simulink model "DataAcquire"  (R2017a)
settings: Solver=FixedStepDiscrete  StartTime=0.0  StopTime=inf  RelTol=1e-3  EnableMultiTasking=on
libraries: simulink x54, stmmbedlib x40
settings Model: SimulationMode=external  ExtModeArchiveFileName=LOGGING  ExtModeArchiveDirName=C:\Users\Salokin\Dropbox\StudiumJobs\Fahrrad Hiwi\STMDISCO  ExtModeAutoIncOneShot=on  Creator=The MathWorks, Inc.  LastModifiedBy=Salokin
settings DataIOCC: LimitDataPoints=on  SaveFormat=Array
settings OptimizationCC: LifeSpan=Inf  MaxStackSize=64
settings DebuggingCC: UnderspecifiedInitializationDetection=Classic  MergeDetectMultiDrivingBlocksExec=none  SolverPrmCheckMsg=warning  AllowSymbolicDim=off  SFUnexpectedBacktrackingDiag=warning  SFNoUnconditionalDefaultTransitionDiag=warning  SFExecutionAtInitializationDiag=none
settings HardwareCC: ProdBitPerPointer=32  ProdBitPerSizeT=32  ProdBitPerPtrDiffT=32  ProdLargestAtomicInteger=Long  ProdLargestAtomicFloat=Double  ProdWordSize=32  ProdHWDeviceType=ARM Compatible->ARM Cortex
settings ModelReferenceCC: PropagateSignalLabelsOutOfModel=off
settings SFSimCC: MATLABDynamicMemAlloc=off
settings RTWCC: SystemTargetFile=ert.tlc  HardwareBoard=STM32F746G-Discovery  TemplateMakefile=ert_default_tmf  Description=Embedded Coder  Toolchain=GNU Tools for ARM Embedded Processors
settings CodeAppCC: IgnoreCustomStorageClasses=off  CustomSymbolStrModelFcn=$N
settings ERTTargetCC: MultiwordLength=2048  ExtMode=on  ExtModeTransport=1  ExtModeMexFile=ext_serial_win32_comm  ExtModeMexArgs=0 28 460800  ConvertIfToSwitch=off  SuppressUnreachableDefaultCases=off
settings ConfigComp: CovMetricSettings=dw  CovHtmlReporting=on  CovSaveCumulativeToWorkspaceVar=on  CovSaveSingleToWorkspaceVar=on  CovExternalEMLEnable=off  CovSFcnEnable=off

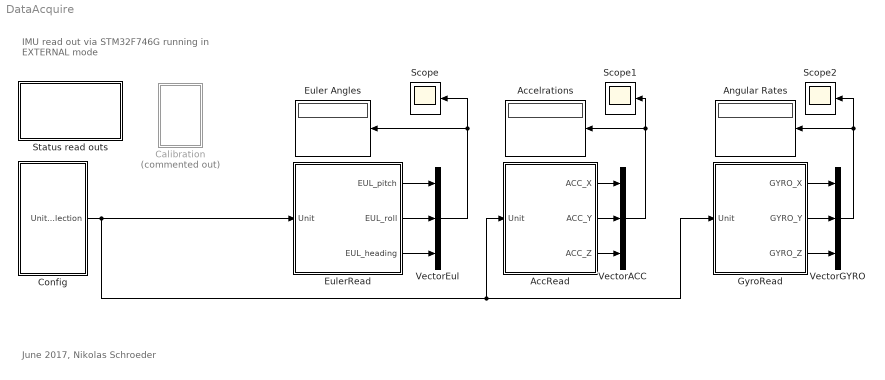
== system DataAcquire ==
  note: June 2017, Nikolas Schroeder
  note: IMU read out via STM32F746G
      | running in EXTERNAL mode
  AccRead : Subsystem
  Accelrations : Display
  Angular Rates : Display
  Calibration : Subsystem  Commented=on
  Config : Subsystem
  Euler Angles : Display
  EulerRead : Subsystem
  GyroRead : Subsystem
  Scope : Scope
  Scope1 : Scope
  Scope2 : Scope
  Status read outs : Subsystem
  VectorACC : Concatenate  NumInputs=3
  VectorEul : Concatenate  NumInputs=3
  VectorGYRO : Concatenate  NumInputs=3
  wires:
  AccRead/1(ACC_X) -> VectorACC/1
  AccRead/2(ACC_Y) -> VectorACC/2
  AccRead/3(ACC_Z) -> VectorACC/3
  GyroRead/1(GYRO_X) -> VectorGYRO/1
  GyroRead/2(GYRO_Y) -> VectorGYRO/2
  GyroRead/3(GYRO_Z) -> VectorGYRO/3
  VectorACC/1 -> Accelrations/1, Scope1/1
  VectorGYRO/1 -> Scope2/1, Angular Rates/1
  EulerRead/1(EUL_pitch) -> VectorEul/1
  EulerRead/2(EUL_roll) -> VectorEul/2
  EulerRead/3(EUL_heading) -> VectorEul/3
  VectorEul/1 -> Scope/1, Euler Angles/1
  Config/1(UnitSelection) -> GyroRead/1(Unit), AccRead/1(Unit), EulerRead/1(Unit)

== system DataAcquire/AccRead ==
  Unit : Inport
  ACCEL_Data_X1_MSB : stmmbedlib/I2C Master Read  I2CModule=0  Mode=Master  SlaveAddress=hex2dec('28')  SlaveByteOrder=BigEndian  Direction=Receiver  RegisterAddressMode=on  RegisterAddress=hex2dec('09')  SlaveDataType=uint8  DataLength=1  NoAck=off  RepeatedStart=off  OutputStatus=on  SampleTime=0.1
  ACCEL_Data_X_LSB : stmmbedlib/I2C Master Read  I2CModule=0  Mode=Master  SlaveAddress=hex2dec('28')  SlaveByteOrder=BigEndian  Direction=Receiver  RegisterAddressMode=on  RegisterAddress=hex2dec('08')  SlaveDataType=uint8  DataLength=1  NoAck=off  RepeatedStart=off  OutputStatus=on  SampleTime=0.1
  ACCEL_Data_Y1_MSB : stmmbedlib/I2C Master Read  I2CModule=0  Mode=Master  SlaveAddress=hex2dec('28')  SlaveByteOrder=BigEndian  Direction=Receiver  RegisterAddressMode=on  RegisterAddress=hex2dec('0B')  SlaveDataType=uint8  DataLength=1  NoAck=off  RepeatedStart=off  OutputStatus=on  SampleTime=0.1
  "ACCEL_Data_Y_LSB " : stmmbedlib/I2C Master Read  I2CModule=0  Mode=Master  SlaveAddress=hex2dec('28')  SlaveByteOrder=BigEndian  Direction=Receiver  RegisterAddressMode=on  RegisterAddress=hex2dec('0A')  SlaveDataType=uint8  DataLength=1  NoAck=off  RepeatedStart=off  OutputStatus=on  SampleTime=0.1
  ACCEL_Data_Z1_MSB : stmmbedlib/I2C Master Read  I2CModule=0  Mode=Master  SlaveAddress=hex2dec('28')  SlaveByteOrder=BigEndian  Direction=Receiver  RegisterAddressMode=on  RegisterAddress=hex2dec('0D')  SlaveDataType=uint8  DataLength=1  NoAck=off  RepeatedStart=off  OutputStatus=on  SampleTime=0.1
  ACCEL_Data_Z_LSB : stmmbedlib/I2C Master Read  I2CModule=0  Mode=Master  SlaveAddress=hex2dec('28')  SlaveByteOrder=BigEndian  Direction=Receiver  RegisterAddressMode=on  RegisterAddress=hex2dec('0C')  SlaveDataType=uint8  DataLength=1  NoAck=off  RepeatedStart=off  OutputStatus=on  SampleTime=0.1
  ACCparserX : Subsystem
  ACCparserY : Subsystem
  ACCparserZ : Subsystem
  Error Status{,1..5} (6 alike) : Display
  ACC_X : Outport
  ACC_Y : Outport  Port=2
  ACC_Z : Outport  Port=3
  wires:
  "ACCEL_Data_Y_LSB "/2 -> Error Status3/1
  ACCEL_Data_Y1_MSB/2 -> Error Status2/1
  ACCEL_Data_Z1_MSB/1 -> ACCparserZ/2(MSB)
  ACCEL_Data_X_LSB/2 -> Error Status/1
  "ACCEL_Data_Y_LSB "/1 -> ACCparserY/1(LSB)
  ACCEL_Data_X1_MSB/2 -> Error Status1/1
  ACCEL_Data_Z_LSB/2 -> Error Status4/1
  ACCEL_Data_Y1_MSB/1 -> ACCparserY/2(MSB)
  ACCEL_Data_Z1_MSB/2 -> Error Status5/1
  ACCEL_Data_Z_LSB/1 -> ACCparserZ/1(LSB)
  Unit/1 -> ACCparserX/3(Unit), ACCparserZ/3(Unit), ACCparserY/3(Unit)
  ACCparserX/1(Out1) -> ACC_X/1
  ACCparserY/1(Out1) -> ACC_Y/1
  ACCEL_Data_X1_MSB/1 -> ACCparserX/2(MSB)
  ACCEL_Data_X_LSB/1 -> ACCparserX/1(LSB)
  ACCparserZ/1(Out1) -> ACC_Z/1

== system DataAcquire/Calibration ==
  Constant{,1..3} (4 alike) : Constant
  I2C Master Write{,1..3} (4 alike) : stmmbedlib/I2C Master Write  I2CModule=0  Mode=Master  SlaveAddress=hex2dec('48')  SlaveByteOrder=BigEndian  Direction=Transmitter  RegisterAddressMode=on  RegisterAddress=uint8(1)  SlaveDataType=uint8  DataLength=2  NoAck=off  RepeatedStart=off  OutputStatus=off
  wires:
  Constant/1 -> I2C Master Write3/1
  Constant2/1 -> I2C Master Write1/1
  Constant3/1 -> I2C Master Write/1
  Constant1/1 -> I2C Master Write2/1

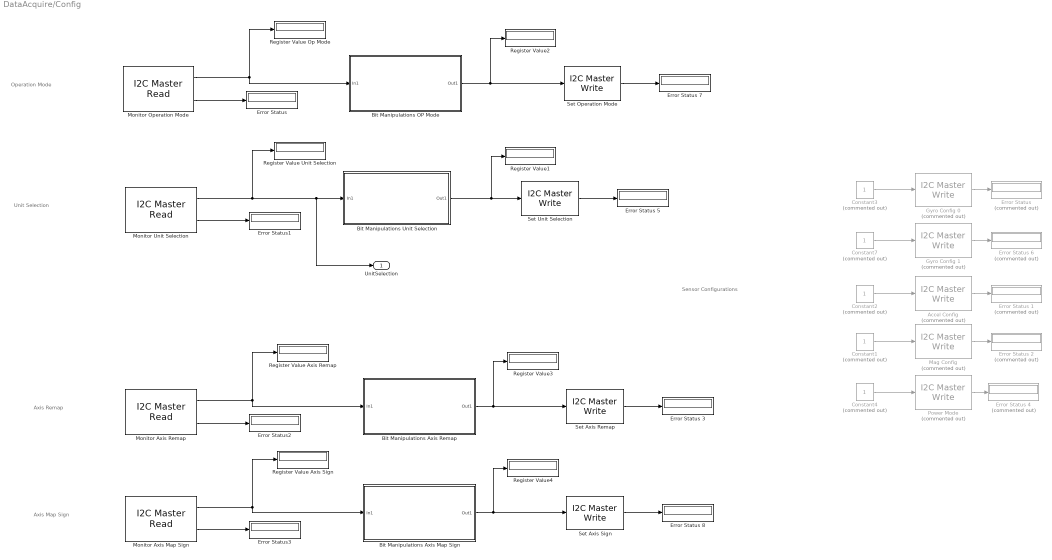
== system DataAcquire/Config ==
  note: Unit Selection
  note: Operation Mode
  note: Sensor Configurations
  note: Axis Remap
  note: Axis Map Sign
  Accel Config : stmmbedlib/I2C Master Write  Commented=on  I2CModule=0  Mode=Master  SlaveAddress=hex2dec('28')  SlaveByteOrder=BigEndian  Direction=Transmitter  RegisterAddressMode=on  RegisterAddress=hex2dec('8')  SlaveDataType=uint8  DataLength=2  NoAck=off  RepeatedStart=off  OutputStatus=on
  Bit Manipulations Axis Map Sign : Subsystem
  Bit Manipulations Axis Remap : Subsystem
  Bit Manipulations OP Mode : Subsystem
  Bit Manipulations Unit Selection : Subsystem
  Constant{1..4,7} (5 alike) : Constant  Commented=on
  Error Status{,1..3} (4 alike) : Display
  Error Status {,1..2,4,6} (5 alike) : Display  Commented=on
  Error Status {3,5,7..8} (4 alike) : Display
  Gyro Config 0 : stmmbedlib/I2C Master Write  Commented=on  I2CModule=0  Mode=Master  SlaveAddress=hex2dec('28')  SlaveByteOrder=BigEndian  Direction=Transmitter  RegisterAddressMode=on  RegisterAddress=hex2dec('A')  SlaveDataType=uint8  DataLength=2  NoAck=off  RepeatedStart=off  OutputStatus=on
  Gyro Config 1 : stmmbedlib/I2C Master Write  Commented=on  I2CModule=0  Mode=Master  SlaveAddress=hex2dec('28')  SlaveByteOrder=BigEndian  Direction=Transmitter  RegisterAddressMode=on  RegisterAddress=hex2dec('B')  SlaveDataType=uint8  DataLength=2  NoAck=off  RepeatedStart=off  OutputStatus=on
  Mag Config : stmmbedlib/I2C Master Write  Commented=on  I2CModule=0  Mode=Master  SlaveAddress=hex2dec('28')  SlaveByteOrder=BigEndian  Direction=Transmitter  RegisterAddressMode=on  RegisterAddress=hex2dec('9')  SlaveDataType=uint8  DataLength=2  NoAck=off  RepeatedStart=off  OutputStatus=on
  Monitor Axis Map Sign : stmmbedlib/I2C Master Read  I2CModule=0  Mode=Master  SlaveAddress=hex2dec('28')  SlaveByteOrder=BigEndian  Direction=Receiver  RegisterAddressMode=on  RegisterAddress=hex2dec('42')  SlaveDataType=uint8  DataLength=1  NoAck=off  RepeatedStart=off  OutputStatus=on  SampleTime=0.1
  Monitor Axis Remap : stmmbedlib/I2C Master Read  I2CModule=0  Mode=Master  SlaveAddress=hex2dec('28')  SlaveByteOrder=BigEndian  Direction=Receiver  RegisterAddressMode=on  RegisterAddress=hex2dec('41')  SlaveDataType=uint8  DataLength=1  NoAck=off  RepeatedStart=off  OutputStatus=on  SampleTime=0.1
  Monitor Operation Mode : stmmbedlib/I2C Master Read  I2CModule=0  Mode=Master  SlaveAddress=hex2dec('28')  SlaveByteOrder=BigEndian  Direction=Receiver  RegisterAddressMode=on  RegisterAddress=hex2dec('3d')  SlaveDataType=uint8  DataLength=1  NoAck=off  RepeatedStart=off  OutputStatus=on  SampleTime=0.01
  Monitor Unit Selection : stmmbedlib/I2C Master Read  I2CModule=0  Mode=Master  SlaveAddress=hex2dec('28')  SlaveByteOrder=BigEndian  Direction=Receiver  RegisterAddressMode=on  RegisterAddress=hex2dec('3b')  SlaveDataType=uint8  DataLength=1  NoAck=off  RepeatedStart=off  OutputStatus=on  SampleTime=0.1
  Power Mode : stmmbedlib/I2C Master Write  Commented=on  I2CModule=0  Mode=Master  SlaveAddress=hex2dec('28')  SlaveByteOrder=BigEndian  Direction=Transmitter  RegisterAddressMode=on  RegisterAddress=hex2dec('3E')  SlaveDataType=uint8  DataLength=2  NoAck=off  RepeatedStart=off  OutputStatus=on
  Register Value Axis Remap : Display
      settings: Format=binary (Stored Integer)
  Register Value Axis Sign : Display
      settings: Format=binary (Stored Integer)
  "Register Value Op Mode " : Display
      settings: Format=binary (Stored Integer)
  Register Value Unit Selection : Display
      settings: Format=binary (Stored Integer)
  Register Value{1..4} (4 alike) : Display
      settings: Format=binary (Stored Integer)
  Set Axis Remap : stmmbedlib/I2C Master Write  I2CModule=0  Mode=Master  SlaveAddress=hex2dec('28')  SlaveByteOrder=BigEndian  Direction=Transmitter  RegisterAddressMode=on  RegisterAddress=hex2dec('41')  SlaveDataType=uint8  DataLength=2  NoAck=off  RepeatedStart=off  OutputStatus=on
  Set Axis Sign : stmmbedlib/I2C Master Write  I2CModule=0  Mode=Master  SlaveAddress=hex2dec('28')  SlaveByteOrder=BigEndian  Direction=Transmitter  RegisterAddressMode=on  RegisterAddress=hex2dec('42')  SlaveDataType=uint8  DataLength=2  NoAck=off  RepeatedStart=off  OutputStatus=on
  Set Operation Mode : stmmbedlib/I2C Master Write  I2CModule=0  Mode=Master  SlaveAddress=hex2dec('28')  SlaveByteOrder=BigEndian  Direction=Transmitter  RegisterAddressMode=on  RegisterAddress=hex2dec('3D')  SlaveDataType=uint8  DataLength=2  NoAck=off  RepeatedStart=off  OutputStatus=on
  Set Unit Selection : stmmbedlib/I2C Master Write  I2CModule=0  Mode=Master  SlaveAddress=hex2dec('28')  SlaveByteOrder=BigEndian  Direction=Transmitter  RegisterAddressMode=on  RegisterAddress=hex2dec('3b')  SlaveDataType=uint8  DataLength=2  NoAck=off  RepeatedStart=off  OutputStatus=on
  UnitSelection : Outport
  wires:
  Constant2/1 -> Accel Config/1
  Constant3/1 -> Gyro Config 0/1
  Constant1/1 -> Mag Config/1
  Constant4/1 -> Power Mode/1
  Gyro Config 0/1 -> "Error Status "/1
  Accel Config/1 -> Error Status 1/1
  Mag Config/1 -> Error Status 2/1
  Power Mode/1 -> Error Status 4/1
  Constant7/1 -> Gyro Config 1/1
  Gyro Config 1/1 -> Error Status 6/1
  Monitor Operation Mode/2 -> Error Status/1
  Monitor Operation Mode/1 -> "Register Value Op Mode "/1, Bit Manipulations OP Mode/1(In1)
  Set Operation Mode/1 -> Error Status 7/1
  Set Unit Selection/1 -> Error Status 5/1
  Monitor Unit Selection/1 -> UnitSelection/1, Bit Manipulations Unit Selection/1(In1), Register Value Unit Selection/1
  Monitor Unit Selection/2 -> Error Status1/1
  Bit Manipulations Unit Selection/1(Out1) -> Register Value1/1, Set Unit Selection/1
  Bit Manipulations OP Mode/1(Out1) -> Register Value2/1, Set Operation Mode/1
  Set Axis Sign/1 -> Error Status 8/1
  Bit Manipulations Axis Remap/1(Out1) -> Register Value3/1, Set Axis Remap/1
  Monitor Axis Remap/1 -> Register Value Axis Remap/1, Bit Manipulations Axis Remap/1(In1)
  Set Axis Remap/1 -> Error Status 3/1
  Monitor Axis Remap/2 -> Error Status2/1
  Monitor Axis Map Sign/1 -> Register Value Axis Sign/1, Bit Manipulations Axis Map Sign/1(In1)
  Monitor Axis Map Sign/2 -> Error Status3/1
  Bit Manipulations Axis Map Sign/1(Out1) -> Register Value4/1, Set Axis Sign/1

== system DataAcquire/EulerRead ==
  Unit : Inport
  EUL_Heading_LSB : stmmbedlib/I2C Master Read  I2CModule=0  Mode=Master  SlaveAddress=hex2dec('28')  SlaveByteOrder=BigEndian  Direction=Receiver  RegisterAddressMode=on  RegisterAddress=hex2dec('1A')  SlaveDataType=uint8  DataLength=1  NoAck=off  RepeatedStart=off  OutputStatus=on  SampleTime=0.1
  EUL_Heading_MSB : stmmbedlib/I2C Master Read  I2CModule=0  Mode=Master  SlaveAddress=hex2dec('28')  SlaveByteOrder=BigEndian  Direction=Receiver  RegisterAddressMode=on  RegisterAddress=hex2dec('1B')  SlaveDataType=uint8  DataLength=1  NoAck=off  RepeatedStart=off  OutputStatus=on  SampleTime=0.1
  "EUL_Pitch_LSB " : stmmbedlib/I2C Master Read  I2CModule=0  Mode=Master  SlaveAddress=hex2dec('28')  SlaveByteOrder=BigEndian  Direction=Receiver  RegisterAddressMode=on  RegisterAddress=hex2dec('1E')  SlaveDataType=uint8  DataLength=1  NoAck=off  RepeatedStart=off  OutputStatus=on  SampleTime=0.1
  "EUL_Pitch_MSB " : stmmbedlib/I2C Master Read  I2CModule=0  Mode=Master  SlaveAddress=hex2dec('28')  SlaveByteOrder=BigEndian  Direction=Receiver  RegisterAddressMode=on  RegisterAddress=hex2dec('1F')  SlaveDataType=uint8  DataLength=1  NoAck=off  RepeatedStart=off  OutputStatus=on  SampleTime=0.1
  "EUL_Roll_LSB " : stmmbedlib/I2C Master Read  I2CModule=0  Mode=Master  SlaveAddress=hex2dec('28')  SlaveByteOrder=BigEndian  Direction=Receiver  RegisterAddressMode=on  RegisterAddress=hex2dec('1C')  SlaveDataType=uint8  DataLength=1  NoAck=off  RepeatedStart=off  OutputStatus=on  SampleTime=0.1
  EUL_Roll_MSB : stmmbedlib/I2C Master Read  I2CModule=0  Mode=Master  SlaveAddress=hex2dec('28')  SlaveByteOrder=BigEndian  Direction=Receiver  RegisterAddressMode=on  RegisterAddress=hex2dec('1D')  SlaveDataType=uint8  DataLength=1  NoAck=off  RepeatedStart=off  OutputStatus=on  SampleTime=0.1
  EULparserHeading : Subsystem
  EULparserPitch : Subsystem
  EULparserRoll : Subsystem
  Error Status{,1..5} (6 alike) : Display
  EUL_pitch : Outport
  EUL_roll : Outport  Port=2
  EUL_heading : Outport  Port=3
  wires:
  EUL_Roll_MSB/2 -> Error Status2/1
  "EUL_Roll_LSB "/2 -> Error Status3/1
  "EUL_Roll_LSB "/1 -> EULparserRoll/1(LSB)
  EUL_Roll_MSB/1 -> EULparserRoll/2(MSB)
  EUL_Heading_MSB/2 -> Error Status5/1
  EUL_Heading_LSB/2 -> Error Status4/1
  EUL_Heading_LSB/1 -> EULparserHeading/1(LSB)
  EUL_Heading_MSB/1 -> EULparserHeading/2(MSB)
  "EUL_Pitch_MSB "/2 -> Error Status1/1
  "EUL_Pitch_MSB "/1 -> EULparserPitch/2(MSB)
  "EUL_Pitch_LSB "/2 -> Error Status/1
  "EUL_Pitch_LSB "/1 -> EULparserPitch/1(LSB)
  Unit/1 -> EULparserPitch/3(Unit), EULparserHeading/3(Unit), EULparserRoll/3(Unit)
  EULparserPitch/1(Out1) -> EUL_pitch/1
  EULparserRoll/1(Out1) -> EUL_roll/1
  EULparserHeading/1(Out1) -> EUL_heading/1

== system DataAcquire/GyroRead ==
  Unit : Inport
  Error Status{,1..5} (6 alike) : Display
  GYROparserX : Subsystem
  GYROparserY : Subsystem
  GYROparserZ : Subsystem
  Gyro_Data_X_LSB : stmmbedlib/I2C Master Read  I2CModule=0  Mode=Master  SlaveAddress=hex2dec('28')  SlaveByteOrder=BigEndian  Direction=Receiver  RegisterAddressMode=on  RegisterAddress=hex2dec('14')  SlaveDataType=uint8  DataLength=1  NoAck=off  RepeatedStart=off  OutputStatus=on  SampleTime=0.1
  Gyro_Data_X_MSB : stmmbedlib/I2C Master Read  I2CModule=0  Mode=Master  SlaveAddress=hex2dec('28')  SlaveByteOrder=BigEndian  Direction=Receiver  RegisterAddressMode=on  RegisterAddress=hex2dec('15')  SlaveDataType=uint8  DataLength=1  NoAck=off  RepeatedStart=off  OutputStatus=on  SampleTime=0.1
  Gyro_Data_Y_LSB : stmmbedlib/I2C Master Read  I2CModule=0  Mode=Master  SlaveAddress=hex2dec('28')  SlaveByteOrder=BigEndian  Direction=Receiver  RegisterAddressMode=on  RegisterAddress=hex2dec('16')  SlaveDataType=uint8  DataLength=1  NoAck=off  RepeatedStart=off  OutputStatus=on  SampleTime=0.1
  Gyro_Data_Y_MSB : stmmbedlib/I2C Master Read  I2CModule=0  Mode=Master  SlaveAddress=hex2dec('28')  SlaveByteOrder=BigEndian  Direction=Receiver  RegisterAddressMode=on  RegisterAddress=hex2dec('17')  SlaveDataType=uint8  DataLength=1  NoAck=off  RepeatedStart=off  OutputStatus=on  SampleTime=0.1
  Gyro_Data_Z_LSB : stmmbedlib/I2C Master Read  I2CModule=0  Mode=Master  SlaveAddress=hex2dec('28')  SlaveByteOrder=BigEndian  Direction=Receiver  RegisterAddressMode=on  RegisterAddress=hex2dec('18')  SlaveDataType=uint8  DataLength=1  NoAck=off  RepeatedStart=off  OutputStatus=on  SampleTime=0.1
  Gyro_Data_Z_MSB : stmmbedlib/I2C Master Read  I2CModule=0  Mode=Master  SlaveAddress=hex2dec('28')  SlaveByteOrder=BigEndian  Direction=Receiver  RegisterAddressMode=on  RegisterAddress=hex2dec('19')  SlaveDataType=uint8  DataLength=1  NoAck=off  RepeatedStart=off  OutputStatus=on  SampleTime=0.1
  GYRO_X : Outport
  GYRO_Y : Outport  Port=2
  GYRO_Z : Outport  Port=3
  wires:
  Gyro_Data_Z_MSB/1 -> GYROparserZ/2(MSB)
  Gyro_Data_X_LSB/2 -> Error Status/1
  Gyro_Data_X_MSB/2 -> Error Status1/1
  Gyro_Data_Z_LSB/2 -> Error Status4/1
  Gyro_Data_Y_LSB/2 -> Error Status3/1
  Gyro_Data_Z_LSB/1 -> GYROparserZ/1(LSB)
  Gyro_Data_Y_MSB/1 -> GYROparserY/2(MSB)
  Gyro_Data_Z_MSB/2 -> Error Status5/1
  Gyro_Data_Y_LSB/1 -> GYROparserY/1(LSB)
  GYROparserY/1(Out1) -> GYRO_Y/1
  Gyro_Data_Y_MSB/2 -> Error Status2/1
  Unit/1 -> GYROparserX/3(Unit), GYROparserZ/3(Unit), GYROparserY/3(Unit)
  GYROparserX/1(Out1) -> GYRO_X/1
  Gyro_Data_X_MSB/1 -> GYROparserX/2(MSB)
  Gyro_Data_X_LSB/1 -> GYROparserX/1(LSB)
  GYROparserZ/1(Out1) -> GYRO_Z/1

== system DataAcquire/Status read outs ==
  note: SYS_STATUS 0x39
      |
      | code (decimal)
      | content
      |
      | 0
      | System idle
      |
      | 1
      | System error
      |
      | 2
      | Initializing perpherals
      |
      | 3
      | System Initialization
      |
      | 4
      | Executing Self Test
      |
      | 5
      | Sensor Fusion Algorithm Running
      |
      | 6
      | System Running without fusion algorithm
  note: CALIB_STAT 0x35: 00 -> not calibrated, 11 -> calibrated
      |
      | bit
      | 7
      | 6
      | 5
      | 4
      | 3
      | 2
      | 1
      | 0
      |
      | content
      | SYS
      | GYRO
      | ACC
      | MAG
  note: ST_Result 0x36: 0 indicates failed Self Test, 1 indicates passed Self Test
      |
      | bit
      | 7 to 4
      | 3
      | 2
      | 1
      | 0
      |
      | content
      | reserved
      | Self Test result MCU
      | Self Test Result GYRO
      | Self Test result MAG
      | Self Test result ACC
  note: SYS_ERROR 0x3A
      |
      | error code (decimal)
      | content
      |
      | 0
      | No error
      |
      | 1
      | Peripheral initialization error
      |
      | 2
      | System initialization error
      |
      | 3
      | Self test result error
      |
      | 4
      | Register Map value out of range
      |
      | 5
      | Register Map address out of range
      |
      | 6
      | Register Map write error
      |
      | 7
      | BNO low power mode not available for selected operation mode
      |
      | 8
      | ACC power mode not available
      |
      | 9
      | Fusion mode configuration error
      |
      | 10
      | Sensor configuration error
  Calibration Status : stmmbedlib/I2C Master Read  Priority=2  I2CModule=0  Mode=Master  SlaveAddress=hex2dec('28')  SlaveByteOrder=BigEndian  Direction=Receiver  RegisterAddressMode=on  RegisterAddress=hex2dec('35')  SlaveDataType=uint8  DataLength=1  NoAck=off  RepeatedStart=off  OutputStatus=on  SampleTime=0.1
  Error Status{,1..4} (5 alike) : Display
  "Read out BNO055 Chip ID " : stmmbedlib/I2C Master Read  Priority=1  I2CModule=0  Mode=Master  SlaveAddress=hex2dec('28')  SlaveByteOrder=BigEndian  Direction=Receiver  RegisterAddressMode=on  RegisterAddress=hex2dec('00')  SlaveDataType=uint8  DataLength=1  NoAck=off  RepeatedStart=off  OutputStatus=on  SampleTime=0.1
  "Read out Self Test Result " : stmmbedlib/I2C Master Read  Priority=2  I2CModule=0  Mode=Master  SlaveAddress=hex2dec('28')  SlaveByteOrder=BigEndian  Direction=Receiver  RegisterAddressMode=on  RegisterAddress=hex2dec('36')  SlaveDataType=uint8  DataLength=1  NoAck=off  RepeatedStart=off  OutputStatus=on  SampleTime=0.1
  Register Value{,1..4} (5 alike) : Display
      Register Value1 settings: Format=binary (Stored Integer)
      Register Value2 settings: Format=binary (Stored Integer)
  SYS Error : stmmbedlib/I2C Master Read  Priority=2  I2CModule=0  Mode=Master  SlaveAddress=hex2dec('28')  SlaveByteOrder=BigEndian  Direction=Receiver  RegisterAddressMode=on  RegisterAddress=hex2dec('3A')  SlaveDataType=uint8  DataLength=1  NoAck=off  RepeatedStart=off  OutputStatus=on  SampleTime=0.1
  Sys Status : stmmbedlib/I2C Master Read  Priority=2  I2CModule=0  Mode=Master  SlaveAddress=hex2dec('28')  SlaveByteOrder=BigEndian  Direction=Receiver  RegisterAddressMode=on  RegisterAddress=hex2dec('39')  SlaveDataType=uint8  DataLength=1  NoAck=off  RepeatedStart=off  OutputStatus=on  SampleTime=0.1
  wires:
  "Read out BNO055 Chip ID "/1 -> Register Value/1
  "Read out Self Test Result "/1 -> Register Value1/1
  "Read out Self Test Result "/2 -> Error Status1/1
  "Read out BNO055 Chip ID "/2 -> Error Status/1
  Calibration Status/1 -> Register Value2/1
  Calibration Status/2 -> Error Status2/1
  Sys Status/2 -> Error Status3/1
  Sys Status/1 -> Register Value3/1
  SYS Error/2 -> Error Status4/1
  SYS Error/1 -> Register Value4/1

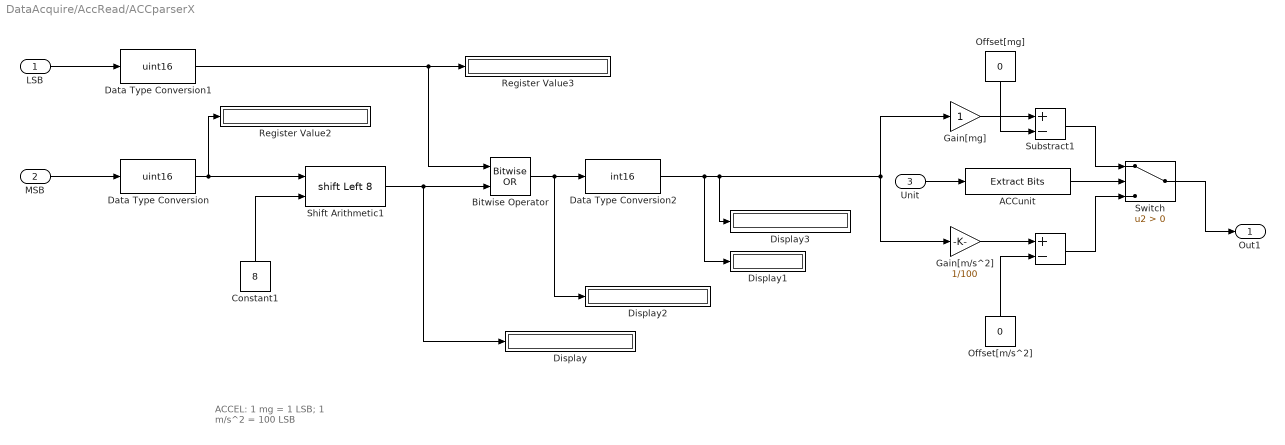
== system DataAcquire/AccRead/ACCparserX ==
  note: ACCEL: 1 mg = 1 LSB; 1 m/s^2 = 100 LSB
  LSB : Inport
  MSB : Inport  Port=2
  Unit : Inport  Port=3
  " " : Sum  Inputs=+-
  ACCunit : simulink/Logic and Bit Operations/Extract Bits  bitsToExtract=Range of bits  numBits=8  bitIdxRange=[0 0]  outScalingMode=Preserve fixed-point scaling
      settings: SourceProductName=Simulink
  Bitwise Operator : simulink/Logic and Bit Operations/Bitwise Operator  logicop=OR  UseBitMask=off  NumInputPorts=2  BitMask=bin2dec('11011001')  BitMaskRealWorld=Stored Integer
  Constant1 : Constant  Value=8
  Data Type Conversion : DataTypeConversion  OutDataTypeStr=uint16
  Data Type Conversion1 : DataTypeConversion  OutDataTypeStr=uint16
  Data Type Conversion2 : DataTypeConversion  OutDataTypeStr=int16
  Display{,1..3} (4 alike) : Display
      Display settings: Format=binary (Stored Integer)
      Display2 settings: Format=binary (Stored Integer)
      Display3 settings: Format=binary (Stored Integer)
  Gain[m/s^2] : Gain  Gain=1/100
  Gain[mg] : Gain
  Offset[m/s^2] : Constant  Value=0
  Offset[mg] : Constant  Value=0
  Register Value2 : Display
      settings: Format=binary (Stored Integer)
  Register Value3 : Display
      settings: Format=binary (Stored Integer)
  Shift Arithmetic1 : ArithShift  BitShiftNumberSource=Input port  BitShiftNumber=8  BitShiftDirection=Left
      settings: InputPortMap=u0,p1
  Substract1 : Sum  Inputs=+-
  Switch : Switch  Criteria=u2 > Threshold
  Out1 : Outport
  wires:
  Substract1/1 -> Switch/1
  Gain[mg]/1 -> Substract1/1
  Offset[mg]/1 -> Substract1/2
  Gain[m/s^2]/1 -> " "/1
  " "/1 -> Switch/3
  Offset[m/s^2]/1 -> " "/2
  Data Type Conversion/1 -> Shift Arithmetic1/1, Register Value2/1
  LSB/1 -> Data Type Conversion1/1
  Data Type Conversion1/1 -> Bitwise Operator/1, Register Value3/1
  Data Type Conversion2/1 -> Gain[mg]/1, Gain[m/s^2]/1, Display3/1, Display1/1
  Shift Arithmetic1/1 -> Display/1, Bitwise Operator/2
  Bitwise Operator/1 -> Display2/1, Data Type Conversion2/1
  Constant1/1 -> Shift Arithmetic1/2
  MSB/1 -> Data Type Conversion/1
  Switch/1 -> Out1/1
  Unit/1 -> ACCunit/1
  ACCunit/1 -> Switch/2

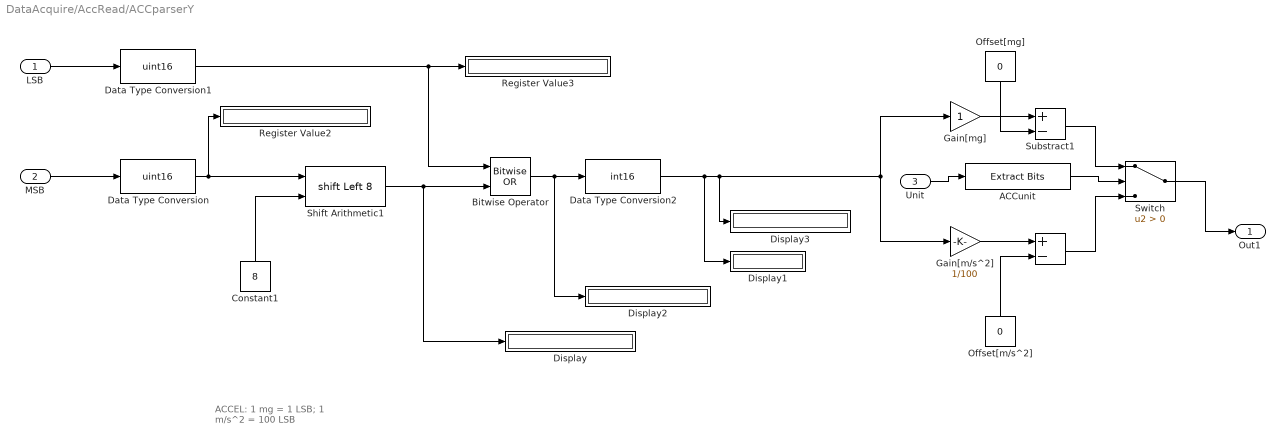
== system DataAcquire/AccRead/ACCparserY ==
  note: ACCEL: 1 mg = 1 LSB; 1 m/s^2 = 100 LSB
  LSB : Inport
  MSB : Inport  Port=2
  Unit : Inport  Port=3
  " " : Sum  Inputs=+-
  ACCunit : simulink/Logic and Bit Operations/Extract Bits  bitsToExtract=Range of bits  numBits=8  bitIdxRange=[0 0]  outScalingMode=Preserve fixed-point scaling
      settings: SourceProductName=Simulink
  Bitwise Operator : simulink/Logic and Bit Operations/Bitwise Operator  logicop=OR  UseBitMask=off  NumInputPorts=2  BitMask=bin2dec('11011001')  BitMaskRealWorld=Stored Integer
  Constant1 : Constant  Value=8
  Data Type Conversion : DataTypeConversion  OutDataTypeStr=uint16
  Data Type Conversion1 : DataTypeConversion  OutDataTypeStr=uint16
  Data Type Conversion2 : DataTypeConversion  OutDataTypeStr=int16
  Display{,1..3} (4 alike) : Display
      Display settings: Format=binary (Stored Integer)
      Display2 settings: Format=binary (Stored Integer)
      Display3 settings: Format=binary (Stored Integer)
  Gain[m/s^2] : Gain  Gain=1/100
  Gain[mg] : Gain
  Offset[m/s^2] : Constant  Value=0
  Offset[mg] : Constant  Value=0
  Register Value2 : Display
      settings: Format=binary (Stored Integer)
  Register Value3 : Display
      settings: Format=binary (Stored Integer)
  Shift Arithmetic1 : ArithShift  BitShiftNumberSource=Input port  BitShiftNumber=8  BitShiftDirection=Left
      settings: InputPortMap=u0,p1
  Substract1 : Sum  Inputs=+-
  Switch : Switch  Criteria=u2 > Threshold
  Out1 : Outport
  wires:
  Substract1/1 -> Switch/1
  Gain[mg]/1 -> Substract1/1
  Offset[mg]/1 -> Substract1/2
  Gain[m/s^2]/1 -> " "/1
  " "/1 -> Switch/3
  Offset[m/s^2]/1 -> " "/2
  Data Type Conversion/1 -> Shift Arithmetic1/1, Register Value2/1
  LSB/1 -> Data Type Conversion1/1
  Data Type Conversion1/1 -> Bitwise Operator/1, Register Value3/1
  Data Type Conversion2/1 -> Gain[mg]/1, Gain[m/s^2]/1, Display3/1, Display1/1
  Shift Arithmetic1/1 -> Display/1, Bitwise Operator/2
  Bitwise Operator/1 -> Display2/1, Data Type Conversion2/1
  Constant1/1 -> Shift Arithmetic1/2
  MSB/1 -> Data Type Conversion/1
  Switch/1 -> Out1/1
  ACCunit/1 -> Switch/2
  Unit/1 -> ACCunit/1

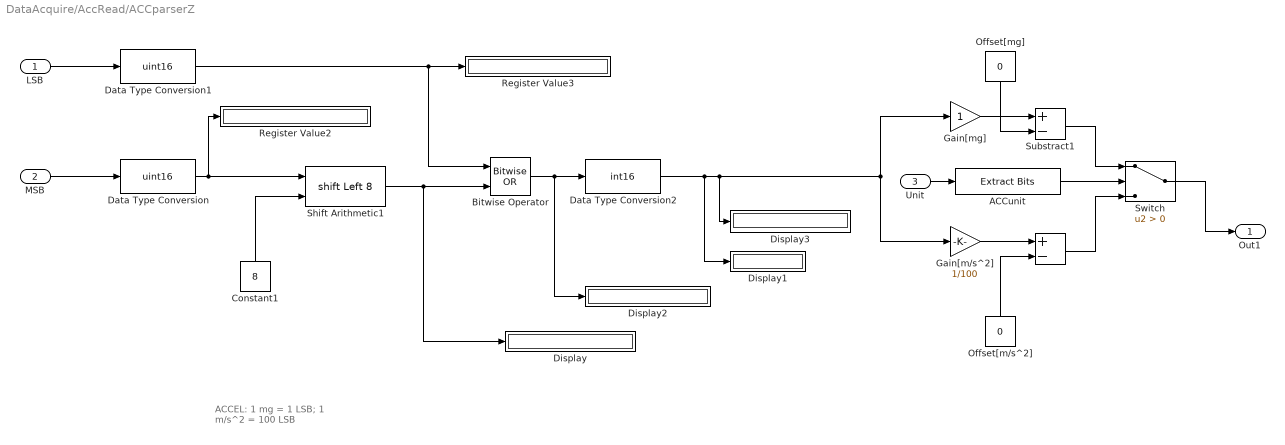
== system DataAcquire/AccRead/ACCparserZ ==
  note: ACCEL: 1 mg = 1 LSB; 1 m/s^2 = 100 LSB
  LSB : Inport
  MSB : Inport  Port=2
  Unit : Inport  Port=3
  " " : Sum  Inputs=+-
  ACCunit : simulink/Logic and Bit Operations/Extract Bits  bitsToExtract=Range of bits  numBits=8  bitIdxRange=[0 0]  outScalingMode=Preserve fixed-point scaling
      settings: SourceProductName=Simulink
  Bitwise Operator : simulink/Logic and Bit Operations/Bitwise Operator  logicop=OR  UseBitMask=off  NumInputPorts=2  BitMask=bin2dec('11011001')  BitMaskRealWorld=Stored Integer
  Constant1 : Constant  Value=8
  Data Type Conversion : DataTypeConversion  OutDataTypeStr=uint16
  Data Type Conversion1 : DataTypeConversion  OutDataTypeStr=uint16
  Data Type Conversion2 : DataTypeConversion  OutDataTypeStr=int16
  Display{,1..3} (4 alike) : Display
      Display settings: Format=binary (Stored Integer)
      Display2 settings: Format=binary (Stored Integer)
      Display3 settings: Format=binary (Stored Integer)
  Gain[m/s^2] : Gain  Gain=1/100
  Gain[mg] : Gain
  Offset[m/s^2] : Constant  Value=0
  Offset[mg] : Constant  Value=0
  Register Value2 : Display
      settings: Format=binary (Stored Integer)
  Register Value3 : Display
      settings: Format=binary (Stored Integer)
  Shift Arithmetic1 : ArithShift  BitShiftNumberSource=Input port  BitShiftNumber=8  BitShiftDirection=Left
      settings: InputPortMap=u0,p1
  Substract1 : Sum  Inputs=+-
  Switch : Switch  Criteria=u2 > Threshold
  Out1 : Outport
  wires:
  Substract1/1 -> Switch/1
  Gain[mg]/1 -> Substract1/1
  Offset[mg]/1 -> Substract1/2
  Gain[m/s^2]/1 -> " "/1
  " "/1 -> Switch/3
  Offset[m/s^2]/1 -> " "/2
  Data Type Conversion/1 -> Shift Arithmetic1/1, Register Value2/1
  LSB/1 -> Data Type Conversion1/1
  Data Type Conversion1/1 -> Bitwise Operator/1, Register Value3/1
  Data Type Conversion2/1 -> Gain[mg]/1, Gain[m/s^2]/1, Display3/1, Display1/1
  Shift Arithmetic1/1 -> Display/1, Bitwise Operator/2
  Bitwise Operator/1 -> Display2/1, Data Type Conversion2/1
  Constant1/1 -> Shift Arithmetic1/2
  MSB/1 -> Data Type Conversion/1
  Switch/1 -> Out1/1
  Unit/1 -> ACCunit/1
  ACCunit/1 -> Switch/2

== system DataAcquire/Config/Bit Manipulations Axis Map Sign ==
  note: value
      | sign
      |
      | 0
      | positive
      |
      | 1
      | negative
  note: bits
      | 7 to 3
      | 2
      | 1
      | 0
      |
      | meaning
      | reserved
      | remapped X-axis sign
      | remapped Y-axis sign
      | remapped Z-axis sign
      |
      | default
      | -
      | 0
      | 0
      | 0
  In1 : Inport
  Clear bit 4 : simulink/Logic and Bit Operations/Bit Clear  iBit=0
      settings: SourceProductName=Simulink  SourceProductBaseCode=SL
  Clear bit 5 : simulink/Logic and Bit Operations/Bit Clear  iBit=1
      settings: SourceProductName=Simulink  SourceProductBaseCode=SL
  Clear bit 6 : simulink/Logic and Bit Operations/Bit Clear  iBit=2
      settings: SourceProductName=Simulink  SourceProductBaseCode=SL
  Manual Switch6 : ManualSwitch  CurrentSetting=0
  Manual Switch7 : ManualSwitch  CurrentSetting=0
  Manual Switch8 : ManualSwitch  CurrentSetting=0
  Set bit 1 : simulink/Logic and Bit Operations/Bit Set  iBit=0
      settings: SourceProductName=Simulink  SourceProductBaseCode=SL
  Set bit 1 1 : simulink/Logic and Bit Operations/Bit Set  iBit=1
      settings: SourceProductName=Simulink  SourceProductBaseCode=SL
  Set bit 4 : simulink/Logic and Bit Operations/Bit Set  iBit=2
      settings: SourceProductName=Simulink  SourceProductBaseCode=SL
  Out1 : Outport
  wires:
  In1/1 -> Clear bit 6/1, Set bit 4/1
  Set bit 1 1/1 -> Manual Switch7/1
  Clear bit 6/1 -> Manual Switch6/2
  Clear bit 5/1 -> Manual Switch7/2
  Manual Switch7/1 -> Clear bit 4/1, Set bit 1/1
  Manual Switch6/1 -> Clear bit 5/1, Set bit 1 1/1
  Clear bit 4/1 -> Manual Switch8/2
  Set bit 1/1 -> Manual Switch8/1
  Set bit 4/1 -> Manual Switch6/1
  Manual Switch8/1 -> Out1/1

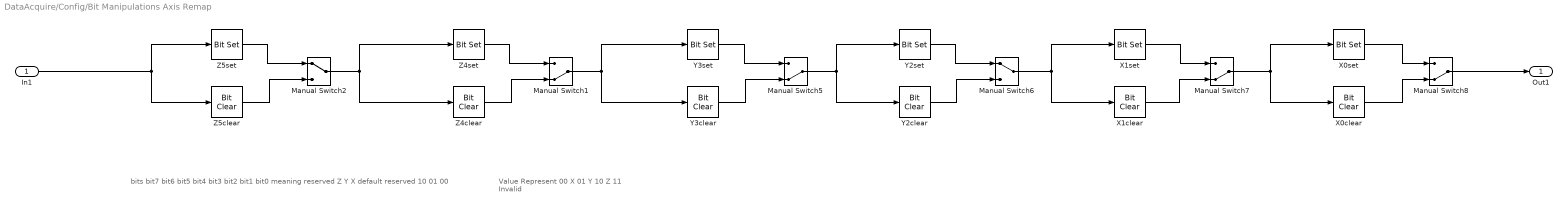
== system DataAcquire/Config/Bit Manipulations Axis Remap ==
  note: Value
      | Represent
      |
      | 00
      | X
      |
      | 01
      | Y
      |
      | 10
      | Z
      |
      | 11
      | Invalid
  note: bits
      | bit7 bit6
      | bit5 bit4
      | bit3 bit2
      | bit1 bit0
      |
      | meaning
      | reserved
      | Z
      | Y
      | X
      |
      | default
      | reserved
      | 10
      | 01
      | 00
  In1 : Inport
  Manual Switch{1,5,7..8} (4 alike) : ManualSwitch  CurrentSetting=0
  Manual Switch2 : ManualSwitch
  Manual Switch6 : ManualSwitch
  X0clear : simulink/Logic and Bit Operations/Bit Clear  iBit=0
      settings: SourceProductName=Simulink  SourceProductBaseCode=SL
  X0set : simulink/Logic and Bit Operations/Bit Set  iBit=0
      settings: SourceProductName=Simulink  SourceProductBaseCode=SL
  X1clear : simulink/Logic and Bit Operations/Bit Clear  iBit=1
      settings: SourceProductName=Simulink  SourceProductBaseCode=SL
  X1set : simulink/Logic and Bit Operations/Bit Set  iBit=1
      settings: SourceProductName=Simulink  SourceProductBaseCode=SL
  Y2clear : simulink/Logic and Bit Operations/Bit Clear  iBit=2
      settings: SourceProductName=Simulink  SourceProductBaseCode=SL
  Y2set : simulink/Logic and Bit Operations/Bit Set  iBit=2
      settings: SourceProductName=Simulink  SourceProductBaseCode=SL
  Y3clear : simulink/Logic and Bit Operations/Bit Clear  iBit=3
      settings: SourceProductName=Simulink  SourceProductBaseCode=SL
  Y3set : simulink/Logic and Bit Operations/Bit Set  iBit=3
      settings: SourceProductName=Simulink  SourceProductBaseCode=SL
  Z4clear : simulink/Logic and Bit Operations/Bit Clear  iBit=4
      settings: SourceProductName=Simulink  SourceProductBaseCode=SL
  Z4set : simulink/Logic and Bit Operations/Bit Set  iBit=4
      settings: SourceProductName=Simulink  SourceProductBaseCode=SL
  Z5clear : simulink/Logic and Bit Operations/Bit Clear  iBit=5
      settings: SourceProductName=Simulink  SourceProductBaseCode=SL
  Z5set : simulink/Logic and Bit Operations/Bit Set  iBit=5
      settings: SourceProductName=Simulink  SourceProductBaseCode=SL
  Out1 : Outport
  wires:
  Manual Switch5/1 -> Y2clear/1, Y2set/1
  X1set/1 -> Manual Switch7/1
  Y3clear/1 -> Manual Switch5/2
  Y2clear/1 -> Manual Switch6/2
  X1clear/1 -> Manual Switch7/2
  Manual Switch7/1 -> X0clear/1, X0set/1
  Manual Switch6/1 -> X1clear/1, X1set/1
  Y3set/1 -> Manual Switch5/1
  X0clear/1 -> Manual Switch8/2
  X0set/1 -> Manual Switch8/1
  Y2set/1 -> Manual Switch6/1
  Manual Switch8/1 -> Out1/1
  Z4set/1 -> Manual Switch1/1
  Z4clear/1 -> Manual Switch1/2
  Manual Switch1/1 -> Y3clear/1, Y3set/1
  Z5set/1 -> Manual Switch2/1
  Z5clear/1 -> Manual Switch2/2
  In1/1 -> Z5clear/1, Z5set/1
  Manual Switch2/1 -> Z4clear/1, Z4set/1

== system DataAcquire/Config/Bit Manipulations OP Mode ==
  note: Mode
      | Name
      | bit3
      | bit2
      | bit1
      | bit0
      |
      | Config
      | Config
      | 0
      | 0
      | 0
      | 0
      |
      | Non Fusion
      | ACCONLY
      | 0
      | 0
      | 0
      | 1
      |
      | Non Fusin
      | MAGONLY
      | 0
      | 0
      | 1
      | 0
      |
      | Non Fusin
      | GYROONLY
      | 0
      | 0
      | 1
      | 1
      |
      | Non Fusion
      | ACCMAG
      | 0
      | 1
      | 0
      | 0
      |
      | Non Fusion
      | ACCGYRO
      | 0
      | 1
      | 0
      | 1
      |
      | Non Fusion
      | MAGGYRO
      | 0
      | 1
      | 1
      | 0
      |
      | Non Fusion
      | AMG
      | 0
      | 1
      | 1
      | 1
      |
      | Fusion
      | IMU
      | 1
      | 0
      | 0
      | 0
      |
      | Fusion
      | COMPASS
      | 1
      | 0
      | 0
      | 1
      |
      | Fusion
      | M4G
      | 1
      | 0
      | 1
      | 0
      |
      | Fusion
      | NDOF_FMC_OFF
      | 1
      | 0
      | 1
      | 1
      |
      | Fusion
      | NDOF
      | 1
      | 1
      | 0
      | 0
  In1 : Inport
  Clear bit 4 : simulink/Logic and Bit Operations/Bit Clear  iBit=0
      settings: SourceProductName=Simulink  SourceProductBaseCode=SL
  Clear bit 5 : simulink/Logic and Bit Operations/Bit Clear  iBit=1
      settings: SourceProductName=Simulink  SourceProductBaseCode=SL
  Clear bit 6 : simulink/Logic and Bit Operations/Bit Clear  iBit=2
      settings: SourceProductName=Simulink  SourceProductBaseCode=SL
  Clear bit 7 : simulink/Logic and Bit Operations/Bit Clear  iBit=3
      settings: SourceProductName=Simulink  SourceProductBaseCode=SL
  Manual Switch5 : ManualSwitch
  Manual Switch6 : ManualSwitch  CurrentSetting=0
  Manual Switch7 : ManualSwitch  CurrentSetting=0
  Manual Switch8 : ManualSwitch  CurrentSetting=0
  Set bit 1 : simulink/Logic and Bit Operations/Bit Set  iBit=0
      settings: SourceProductName=Simulink  SourceProductBaseCode=SL
  Set bit 1 1 : simulink/Logic and Bit Operations/Bit Set  iBit=1
      settings: SourceProductName=Simulink  SourceProductBaseCode=SL
  Set bit 4 : simulink/Logic and Bit Operations/Bit Set  iBit=2
      settings: SourceProductName=Simulink  SourceProductBaseCode=SL
  Set bit 5 : simulink/Logic and Bit Operations/Bit Set  iBit=3
      settings: SourceProductName=Simulink  SourceProductBaseCode=SL
  Out1 : Outport
  wires:
  Manual Switch5/1 -> Clear bit 6/1, Set bit 4/1
  Set bit 1 1/1 -> Manual Switch7/1
  Clear bit 7/1 -> Manual Switch5/2
  Clear bit 6/1 -> Manual Switch6/2
  Clear bit 5/1 -> Manual Switch7/2
  Manual Switch7/1 -> Clear bit 4/1, Set bit 1/1
  Manual Switch6/1 -> Clear bit 5/1, Set bit 1 1/1
  Set bit 5/1 -> Manual Switch5/1
  Clear bit 4/1 -> Manual Switch8/2
  Set bit 1/1 -> Manual Switch8/1
  Set bit 4/1 -> Manual Switch6/1
  In1/1 -> Clear bit 7/1, Set bit 5/1
  Manual Switch8/1 -> Out1/1

== system DataAcquire/Config/Bit Manipulations Unit Selection ==
  In1 : Inport
  ACCEL Gravity Vector [mg] : simulink/Logic and Bit Operations/Bit Set  iBit=0
      settings: SourceProductName=Simulink  SourceProductBaseCode=SL
  ACCEL linear [m/s^2] : simulink/Logic and Bit Operations/Bit Clear  iBit=0
      settings: SourceProductName=Simulink  SourceProductBaseCode=SL
  Android : simulink/Logic and Bit Operations/Bit Set  iBit=7
      settings: SourceProductName=Simulink  SourceProductBaseCode=SL
  Angular Rate [Dps] : simulink/Logic and Bit Operations/Bit Clear  iBit=1
      settings: SourceProductName=Simulink  SourceProductBaseCode=SL
  Angular Rate [Rps] : simulink/Logic and Bit Operations/Bit Set  iBit=1
      settings: SourceProductName=Simulink  SourceProductBaseCode=SL
  EULER [deg] : simulink/Logic and Bit Operations/Bit Clear  iBit=2
      settings: SourceProductName=Simulink  SourceProductBaseCode=SL
  EULER [rad] : simulink/Logic and Bit Operations/Bit Set  iBit=2
      settings: SourceProductName=Simulink  SourceProductBaseCode=SL
  Manual Switch{,1..4} (5 alike) : ManualSwitch  CurrentSetting=0
  Temp [°C] : simulink/Logic and Bit Operations/Bit Clear  iBit=4
      settings: SourceProductName=Simulink  SourceProductBaseCode=SL
  Temp [°F] : simulink/Logic and Bit Operations/Bit Set  iBit=4
      settings: SourceProductName=Simulink  SourceProductBaseCode=SL
  Windows : simulink/Logic and Bit Operations/Bit Clear  iBit=7
      settings: SourceProductName=Simulink  SourceProductBaseCode=SL
  Out1 : Outport
  wires:
  EULER [deg]/1 -> Manual Switch2/2
  Manual Switch1/1 -> EULER [deg]/1, EULER [rad]/1
  EULER [rad]/1 -> Manual Switch2/1
  Angular Rate [Dps]/1 -> Manual Switch3/2
  Angular Rate [Rps]/1 -> Manual Switch3/1
  Manual Switch2/1 -> Angular Rate [Dps]/1, Angular Rate [Rps]/1
  Manual Switch/1 -> Temp [°C]/1, Temp [°F]/1
  Windows/1 -> Manual Switch/2
  Temp [°C]/1 -> Manual Switch1/2
  Temp [°F]/1 -> Manual Switch1/1
  Manual Switch3/1 -> ACCEL linear [m/s^2]/1, ACCEL Gravity Vector [mg]/1
  ACCEL Gravity Vector [mg]/1 -> Manual Switch4/1
  ACCEL linear [m/s^2]/1 -> Manual Switch4/2
  Android/1 -> Manual Switch/1
  In1/1 -> Windows/1, Android/1
  Manual Switch4/1 -> Out1/1

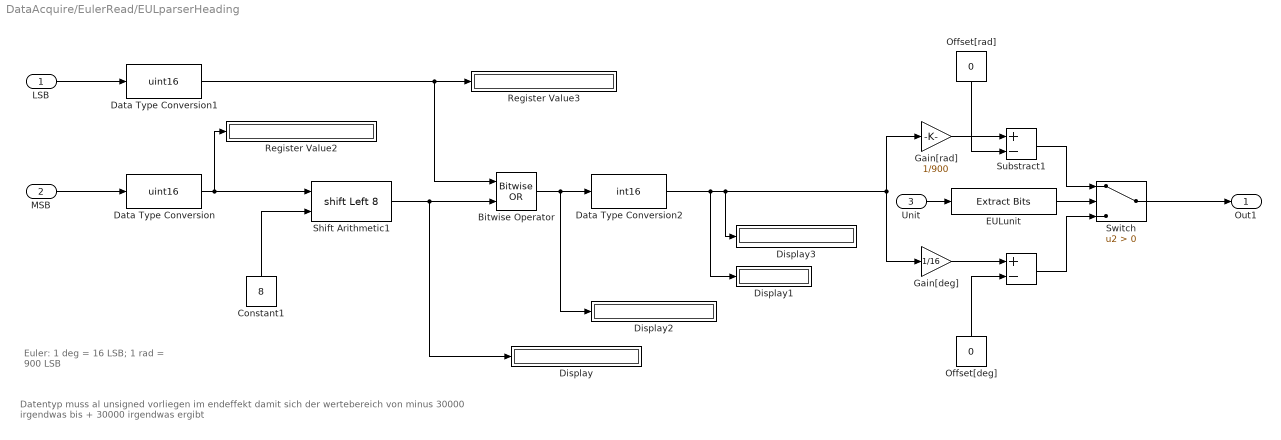
== system DataAcquire/EulerRead/EULparserHeading ==
  note: Datentyp muss al unsigned vorliegen im endeffekt damit sich der wertebereich von minus 30000 irgendwas bis + 30000 irgendwas ergibt
  note: Euler: 1 deg = 16 LSB; 1 rad = 900 LSB
  LSB : Inport
  MSB : Inport  Port=2
  Unit : Inport  Port=3
  " " : Sum  Inputs=+-
  Bitwise Operator : simulink/Logic and Bit Operations/Bitwise Operator  logicop=OR  UseBitMask=off  NumInputPorts=2  BitMask=bin2dec('11011001')  BitMaskRealWorld=Stored Integer
  Constant1 : Constant  Value=8
  Data Type Conversion : DataTypeConversion  OutDataTypeStr=uint16
  Data Type Conversion1 : DataTypeConversion  OutDataTypeStr=uint16
  Data Type Conversion2 : DataTypeConversion  OutDataTypeStr=int16
  Display{,1..3} (4 alike) : Display
      Display settings: Format=binary (Stored Integer)
      Display2 settings: Format=binary (Stored Integer)
      Display3 settings: Format=binary (Stored Integer)
  EULunit : simulink/Logic and Bit Operations/Extract Bits  bitsToExtract=Range of bits  numBits=8  bitIdxRange=[2 2]  outScalingMode=Preserve fixed-point scaling
      settings: SourceProductName=Simulink
  Gain[deg] : Gain  Gain=1/16
  Gain[rad] : Gain  Gain=1/900
  Offset[deg] : Constant  Value=0
  Offset[rad] : Constant  Value=0
  Register Value2 : Display
      settings: Format=binary (Stored Integer)
  Register Value3 : Display
      settings: Format=binary (Stored Integer)
  Shift Arithmetic1 : ArithShift  BitShiftNumberSource=Input port  BitShiftNumber=8  BitShiftDirection=Left
      settings: InputPortMap=u0,p1
  Substract1 : Sum  Inputs=+-
  Switch : Switch  Criteria=u2 > Threshold
  Out1 : Outport
  wires:
  Shift Arithmetic1/1 -> Display/1, Bitwise Operator/2
  Constant1/1 -> Shift Arithmetic1/2
  Gain[deg]/1 -> " "/1
  Gain[rad]/1 -> Substract1/1
  Substract1/1 -> Switch/1
  Offset[deg]/1 -> " "/2
  Bitwise Operator/1 -> Display2/1, Data Type Conversion2/1
  Switch/1 -> Out1/1
  " "/1 -> Switch/3
  Offset[rad]/1 -> Substract1/2
  MSB/1 -> Data Type Conversion/1
  Data Type Conversion/1 -> Shift Arithmetic1/1, Register Value2/1
  LSB/1 -> Data Type Conversion1/1
  Data Type Conversion1/1 -> Bitwise Operator/1, Register Value3/1
  Data Type Conversion2/1 -> Gain[deg]/1, Gain[rad]/1, Display3/1, Display1/1
  Unit/1 -> EULunit/1
  EULunit/1 -> Switch/2

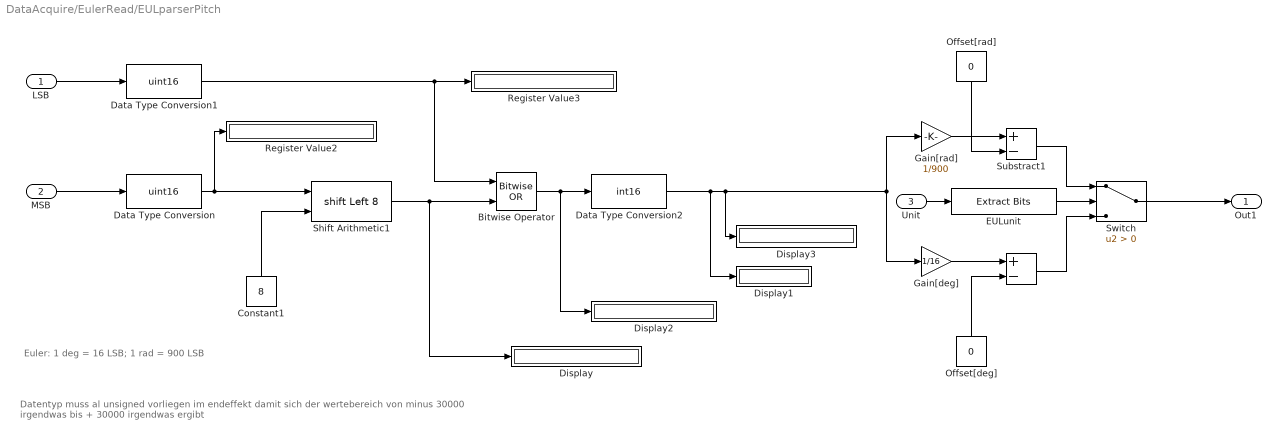
== system DataAcquire/EulerRead/EULparserPitch ==
  note: Datentyp muss al unsigned vorliegen im endeffekt damit sich der wertebereich von minus 30000 irgendwas bis + 30000 irgendwas ergibt
  note: Euler: 1 deg = 16 LSB; 1 rad = 900 LSB
  LSB : Inport
  MSB : Inport  Port=2
  Unit : Inport  Port=3
  " " : Sum  Inputs=+-
  Bitwise Operator : simulink/Logic and Bit Operations/Bitwise Operator  logicop=OR  UseBitMask=off  NumInputPorts=2  BitMask=bin2dec('11011001')  BitMaskRealWorld=Stored Integer
  Constant1 : Constant  Value=8
  Data Type Conversion : DataTypeConversion  OutDataTypeStr=uint16
  Data Type Conversion1 : DataTypeConversion  OutDataTypeStr=uint16
  Data Type Conversion2 : DataTypeConversion  OutDataTypeStr=int16
  Display{,1..3} (4 alike) : Display
      Display settings: Format=binary (Stored Integer)
      Display2 settings: Format=binary (Stored Integer)
      Display3 settings: Format=binary (Stored Integer)
  EULunit : simulink/Logic and Bit Operations/Extract Bits  bitsToExtract=Range of bits  numBits=8  bitIdxRange=[2 2]  outScalingMode=Preserve fixed-point scaling
      settings: SourceProductName=Simulink
  Gain[deg] : Gain  Gain=1/16
  Gain[rad] : Gain  Gain=1/900
  Offset[deg] : Constant  Value=0
  Offset[rad] : Constant  Value=0
  Register Value2 : Display
      settings: Format=binary (Stored Integer)
  Register Value3 : Display
      settings: Format=binary (Stored Integer)
  Shift Arithmetic1 : ArithShift  BitShiftNumberSource=Input port  BitShiftNumber=8  BitShiftDirection=Left
      settings: InputPortMap=u0,p1
  Substract1 : Sum  Inputs=+-
  Switch : Switch  Criteria=u2 > Threshold
  Out1 : Outport
  wires:
  Shift Arithmetic1/1 -> Display/1, Bitwise Operator/2
  Constant1/1 -> Shift Arithmetic1/2
  Gain[deg]/1 -> " "/1
  Gain[rad]/1 -> Substract1/1
  Substract1/1 -> Switch/1
  Offset[deg]/1 -> " "/2
  Bitwise Operator/1 -> Display2/1, Data Type Conversion2/1
  Switch/1 -> Out1/1
  " "/1 -> Switch/3
  Offset[rad]/1 -> Substract1/2
  MSB/1 -> Data Type Conversion/1
  Data Type Conversion/1 -> Shift Arithmetic1/1, Register Value2/1
  LSB/1 -> Data Type Conversion1/1
  Data Type Conversion1/1 -> Bitwise Operator/1, Register Value3/1
  Data Type Conversion2/1 -> Gain[deg]/1, Gain[rad]/1, Display3/1, Display1/1
  Unit/1 -> EULunit/1
  EULunit/1 -> Switch/2

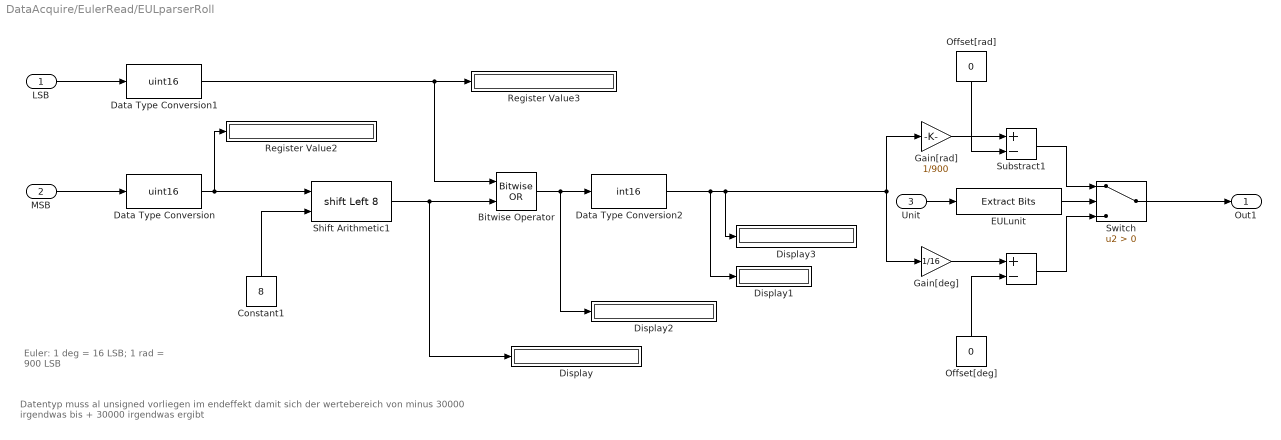
== system DataAcquire/EulerRead/EULparserRoll ==
  note: Datentyp muss al unsigned vorliegen im endeffekt damit sich der wertebereich von minus 30000 irgendwas bis + 30000 irgendwas ergibt
  note: Euler: 1 deg = 16 LSB; 1 rad = 900 LSB
  LSB : Inport
  MSB : Inport  Port=2
  Unit : Inport  Port=3
  " " : Sum  Inputs=+-
  Bitwise Operator : simulink/Logic and Bit Operations/Bitwise Operator  logicop=OR  UseBitMask=off  NumInputPorts=2  BitMask=bin2dec('11011001')  BitMaskRealWorld=Stored Integer
  Constant1 : Constant  Value=8
  Data Type Conversion : DataTypeConversion  OutDataTypeStr=uint16
  Data Type Conversion1 : DataTypeConversion  OutDataTypeStr=uint16
  Data Type Conversion2 : DataTypeConversion  OutDataTypeStr=int16
  Display{,1..3} (4 alike) : Display
      Display settings: Format=binary (Stored Integer)
      Display2 settings: Format=binary (Stored Integer)
      Display3 settings: Format=binary (Stored Integer)
  EULunit : simulink/Logic and Bit Operations/Extract Bits  bitsToExtract=Range of bits  numBits=8  bitIdxRange=[2 2]  outScalingMode=Preserve fixed-point scaling
      settings: SourceProductName=Simulink
  Gain[deg] : Gain  Gain=1/16
  Gain[rad] : Gain  Gain=1/900
  Offset[deg] : Constant  Value=0
  Offset[rad] : Constant  Value=0
  Register Value2 : Display
      settings: Format=binary (Stored Integer)
  Register Value3 : Display
      settings: Format=binary (Stored Integer)
  Shift Arithmetic1 : ArithShift  BitShiftNumberSource=Input port  BitShiftNumber=8  BitShiftDirection=Left
      settings: InputPortMap=u0,p1
  Substract1 : Sum  Inputs=+-
  Switch : Switch  Criteria=u2 > Threshold
  Out1 : Outport
  wires:
  Shift Arithmetic1/1 -> Display/1, Bitwise Operator/2
  Constant1/1 -> Shift Arithmetic1/2
  Gain[deg]/1 -> " "/1
  Gain[rad]/1 -> Substract1/1
  Substract1/1 -> Switch/1
  Offset[deg]/1 -> " "/2
  Bitwise Operator/1 -> Display2/1, Data Type Conversion2/1
  Switch/1 -> Out1/1
  " "/1 -> Switch/3
  Offset[rad]/1 -> Substract1/2
  MSB/1 -> Data Type Conversion/1
  Data Type Conversion/1 -> Shift Arithmetic1/1, Register Value2/1
  LSB/1 -> Data Type Conversion1/1
  Data Type Conversion1/1 -> Bitwise Operator/1, Register Value3/1
  Data Type Conversion2/1 -> Gain[deg]/1, Gain[rad]/1, Display3/1, Display1/1
  Unit/1 -> EULunit/1
  EULunit/1 -> Switch/2

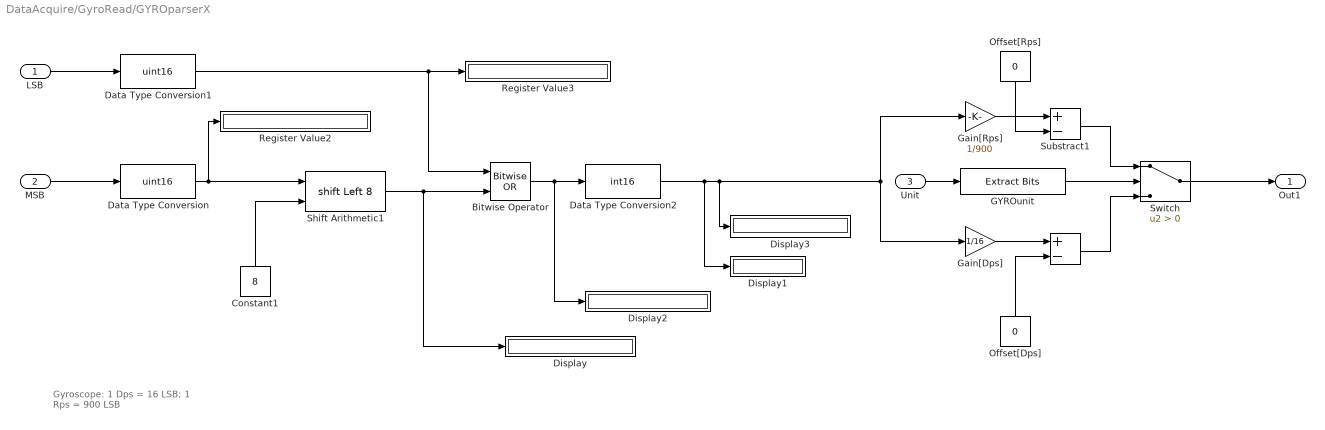
== system DataAcquire/GyroRead/GYROparserX ==
  note: Gyroscope: 1 Dps = 16 LSB; 1 Rps = 900 LSB
  LSB : Inport
  MSB : Inport  Port=2
  Unit : Inport  Port=3
  " " : Sum  Inputs=+-
  Bitwise Operator : simulink/Logic and Bit Operations/Bitwise Operator  logicop=OR  UseBitMask=off  NumInputPorts=2  BitMask=bin2dec('11011001')  BitMaskRealWorld=Stored Integer
  Constant1 : Constant  Value=8
  Data Type Conversion : DataTypeConversion  OutDataTypeStr=uint16
  Data Type Conversion1 : DataTypeConversion  OutDataTypeStr=uint16
  Data Type Conversion2 : DataTypeConversion  OutDataTypeStr=int16
  Display{,1..3} (4 alike) : Display
      Display settings: Format=binary (Stored Integer)
      Display2 settings: Format=binary (Stored Integer)
      Display3 settings: Format=binary (Stored Integer)
  GYROunit : simulink/Logic and Bit Operations/Extract Bits  bitsToExtract=Range of bits  numBits=8  bitIdxRange=[1 1]  outScalingMode=Preserve fixed-point scaling
      settings: SourceProductName=Simulink
  Gain[Dps] : Gain  Gain=1/16
  Gain[Rps] : Gain  Gain=1/900
  Offset[Dps] : Constant  Value=0
  Offset[Rps] : Constant  Value=0
  Register Value2 : Display
      settings: Format=binary (Stored Integer)
  Register Value3 : Display
      settings: Format=binary (Stored Integer)
  Shift Arithmetic1 : ArithShift  BitShiftNumberSource=Input port  BitShiftNumber=8  BitShiftDirection=Left
      settings: InputPortMap=u0,p1
  Substract1 : Sum  Inputs=+-
  Switch : Switch  Criteria=u2 > Threshold
  Out1 : Outport
  wires:
  Gain[Dps]/1 -> " "/1
  Gain[Rps]/1 -> Substract1/1
  Substract1/1 -> Switch/1
  Offset[Dps]/1 -> " "/2
  Switch/1 -> Out1/1
  " "/1 -> Switch/3
  Offset[Rps]/1 -> Substract1/2
  MSB/1 -> Data Type Conversion/1
  Constant1/1 -> Shift Arithmetic1/2
  Bitwise Operator/1 -> Display2/1, Data Type Conversion2/1
  Shift Arithmetic1/1 -> Display/1, Bitwise Operator/2
  Data Type Conversion1/1 -> Bitwise Operator/1, Register Value3/1
  Data Type Conversion/1 -> Shift Arithmetic1/1, Register Value2/1
  LSB/1 -> Data Type Conversion1/1
  Data Type Conversion2/1 -> Gain[Dps]/1, Gain[Rps]/1, Display3/1, Display1/1
  GYROunit/1 -> Switch/2
  Unit/1 -> GYROunit/1

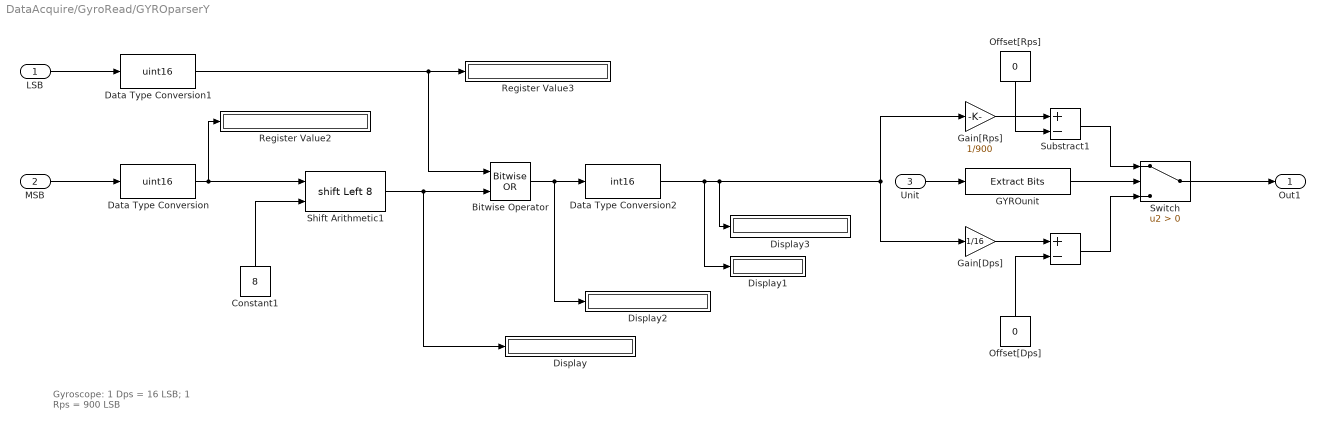
== system DataAcquire/GyroRead/GYROparserY ==
  note: Gyroscope: 1 Dps = 16 LSB; 1 Rps = 900 LSB
  LSB : Inport
  MSB : Inport  Port=2
  Unit : Inport  Port=3
  " " : Sum  Inputs=+-
  Bitwise Operator : simulink/Logic and Bit Operations/Bitwise Operator  logicop=OR  UseBitMask=off  NumInputPorts=2  BitMask=bin2dec('11011001')  BitMaskRealWorld=Stored Integer
  Constant1 : Constant  Value=8
  Data Type Conversion : DataTypeConversion  OutDataTypeStr=uint16
  Data Type Conversion1 : DataTypeConversion  OutDataTypeStr=uint16
  Data Type Conversion2 : DataTypeConversion  OutDataTypeStr=int16
  Display{,1..3} (4 alike) : Display
      Display settings: Format=binary (Stored Integer)
      Display2 settings: Format=binary (Stored Integer)
      Display3 settings: Format=binary (Stored Integer)
  GYROunit : simulink/Logic and Bit Operations/Extract Bits  bitsToExtract=Range of bits  numBits=8  bitIdxRange=[1 1]  outScalingMode=Preserve fixed-point scaling
      settings: SourceProductName=Simulink
  Gain[Dps] : Gain  Gain=1/16
  Gain[Rps] : Gain  Gain=1/900
  Offset[Dps] : Constant  Value=0
  Offset[Rps] : Constant  Value=0
  Register Value2 : Display
      settings: Format=binary (Stored Integer)
  Register Value3 : Display
      settings: Format=binary (Stored Integer)
  Shift Arithmetic1 : ArithShift  BitShiftNumberSource=Input port  BitShiftNumber=8  BitShiftDirection=Left
      settings: InputPortMap=u0,p1
  Substract1 : Sum  Inputs=+-
  Switch : Switch  Criteria=u2 > Threshold
  Out1 : Outport
  wires:
  Gain[Dps]/1 -> " "/1
  Gain[Rps]/1 -> Substract1/1
  Substract1/1 -> Switch/1
  Offset[Dps]/1 -> " "/2
  Switch/1 -> Out1/1
  " "/1 -> Switch/3
  Offset[Rps]/1 -> Substract1/2
  MSB/1 -> Data Type Conversion/1
  Constant1/1 -> Shift Arithmetic1/2
  Bitwise Operator/1 -> Display2/1, Data Type Conversion2/1
  Shift Arithmetic1/1 -> Display/1, Bitwise Operator/2
  Data Type Conversion1/1 -> Bitwise Operator/1, Register Value3/1
  Data Type Conversion/1 -> Shift Arithmetic1/1, Register Value2/1
  LSB/1 -> Data Type Conversion1/1
  Data Type Conversion2/1 -> Gain[Dps]/1, Gain[Rps]/1, Display3/1, Display1/1
  Unit/1 -> GYROunit/1
  GYROunit/1 -> Switch/2

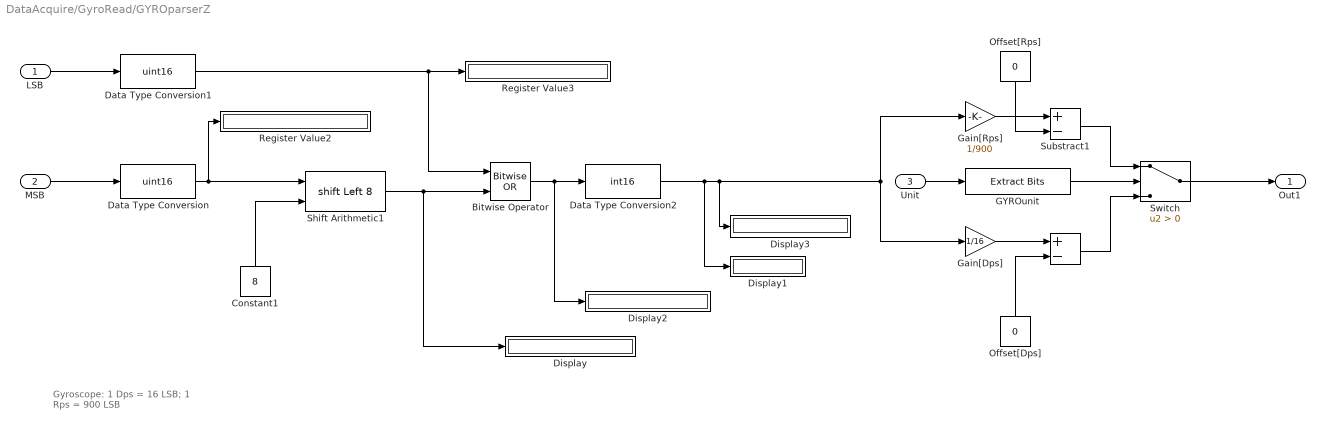
== system DataAcquire/GyroRead/GYROparserZ ==
  note: Gyroscope: 1 Dps = 16 LSB; 1 Rps = 900 LSB
  LSB : Inport
  MSB : Inport  Port=2
  Unit : Inport  Port=3
  " " : Sum  Inputs=+-
  Bitwise Operator : simulink/Logic and Bit Operations/Bitwise Operator  logicop=OR  UseBitMask=off  NumInputPorts=2  BitMask=bin2dec('11011001')  BitMaskRealWorld=Stored Integer
  Constant1 : Constant  Value=8
  Data Type Conversion : DataTypeConversion  OutDataTypeStr=uint16
  Data Type Conversion1 : DataTypeConversion  OutDataTypeStr=uint16
  Data Type Conversion2 : DataTypeConversion  OutDataTypeStr=int16
  Display{,1..3} (4 alike) : Display
      Display settings: Format=binary (Stored Integer)
      Display2 settings: Format=binary (Stored Integer)
      Display3 settings: Format=binary (Stored Integer)
  GYROunit : simulink/Logic and Bit Operations/Extract Bits  bitsToExtract=Range of bits  numBits=8  bitIdxRange=[1 1]  outScalingMode=Preserve fixed-point scaling
      settings: SourceProductName=Simulink
  Gain[Dps] : Gain  Gain=1/16
  Gain[Rps] : Gain  Gain=1/900
  Offset[Dps] : Constant  Value=0
  Offset[Rps] : Constant  Value=0
  Register Value2 : Display
      settings: Format=binary (Stored Integer)
  Register Value3 : Display
      settings: Format=binary (Stored Integer)
  Shift Arithmetic1 : ArithShift  BitShiftNumberSource=Input port  BitShiftNumber=8  BitShiftDirection=Left
      settings: InputPortMap=u0,p1
  Substract1 : Sum  Inputs=+-
  Switch : Switch  Criteria=u2 > Threshold
  Out1 : Outport
  wires:
  Gain[Dps]/1 -> " "/1
  Gain[Rps]/1 -> Substract1/1
  Substract1/1 -> Switch/1
  Offset[Dps]/1 -> " "/2
  Switch/1 -> Out1/1
  " "/1 -> Switch/3
  Offset[Rps]/1 -> Substract1/2
  MSB/1 -> Data Type Conversion/1
  Constant1/1 -> Shift Arithmetic1/2
  Bitwise Operator/1 -> Display2/1, Data Type Conversion2/1
  Shift Arithmetic1/1 -> Display/1, Bitwise Operator/2
  Data Type Conversion1/1 -> Bitwise Operator/1, Register Value3/1
  Data Type Conversion/1 -> Shift Arithmetic1/1, Register Value2/1
  LSB/1 -> Data Type Conversion1/1
  Data Type Conversion2/1 -> Gain[Dps]/1, Gain[Rps]/1, Display3/1, Display1/1
  GYROunit/1 -> Switch/2
  Unit/1 -> GYROunit/1
